simulink library "halout"  (R2021b)
settings: Solver=VariableStepAuto  StartTime=0.0  StopTime=10.0  RelTol=1e-3
undefined symbols (not defined in the file): C_TASK_5MS_S, FALSE, KHAL_CAN1TxReq_flg, KHAL_CAN2TxReq_flg, KHAL_CAN3FD3VCU1toNIDECTxReq_flg, KHAL_CAN3FD3VCU1TxReq_flg, KHAL_CAN3FD3VCU2E2E_flg, KHAL_CAN3FD3VCU2toNIDECE2E_flg, KHAL_CAN3FD3VCU2toNIDECTxReq_flg, KHAL_CAN3FD3VCU2TxReq_flg, KHAL_CAN3TxReq_flg, KHAL_CAN4FD4CE1000E2E_flg, KHAL_CAN4FD4CE1000TxReq_flg, KHAL_CAN4TxReq_flg, KHAL_CAN5TxReq_flg, KHAL_CAN7TxReq_flg, ONE_INT, TRUE, ZERO_INT
libraries: FVT_lib x258, simulink x115
(part 16 of 17)

== system halout/HAL_OUT/CAN4/FD4_CE200_0_0x217/AmbLightColor4 ==
  AmbLightColor4 : Inport
  Data Type Conversion : DataTypeConversion  OutDataTypeStr=uint8  RndMeth=Round
  CAN4_AmbLightColor4 : Outport
  wires:
  Data Type Conversion/1 -> CAN4_AmbLightColor4/1
  AmbLightColor4/1 -> Data Type Conversion/1

== system halout/HAL_OUT/CAN4/FD4_CE200_0_0x217/AmbLightColor5 ==
  AmbLightColor5 : Inport
  Data Type Conversion : DataTypeConversion  OutDataTypeStr=uint8  RndMeth=Round
  CAN4_AmbLightColor5 : Outport
  wires:
  Data Type Conversion/1 -> CAN4_AmbLightColor5/1
  AmbLightColor5/1 -> Data Type Conversion/1

== system halout/HAL_OUT/CAN4/FD4_CE200_0_0x217/AmbLightColor6 ==
  AmbLightColor6 : Inport
  Data Type Conversion : DataTypeConversion  OutDataTypeStr=uint8  RndMeth=Round
  CAN4_AmbLightColor6 : Outport
  wires:
  Data Type Conversion/1 -> CAN4_AmbLightColor6/1
  AmbLightColor6/1 -> Data Type Conversion/1

== system halout/HAL_OUT/CAN4/FD4_CE200_0_0x217/BCMBuzzerReq ==
  BCMBuzzerReq : Inport
  Data Type Conversion : DataTypeConversion  OutDataTypeStr=uint8  RndMeth=Round
  CAN4_BCM_Buzzer_Req : Outport
  wires:
  Data Type Conversion/1 -> CAN4_BCM_Buzzer_Req/1
  BCMBuzzerReq/1 -> Data Type Conversion/1

== system halout/HAL_OUT/CAN4/FD4_CE200_0_0x217/FDCBCMATCtrlCmd ==
  FDCBCMATCtrlCmd : Inport
  Data Type Conversion : DataTypeConversion  OutDataTypeStr=uint8  RndMeth=Round
  CAN4_FDC_BCM_ATCtrl_Cmd : Outport
  wires:
  Data Type Conversion/1 -> CAN4_FDC_BCM_ATCtrl_Cmd/1
  FDCBCMATCtrlCmd/1 -> Data Type Conversion/1

== system halout/HAL_OUT/CAN4/FD4_CE200_0_0x217/FDCBCMDimSw ==
  FDCBCMDimSw : Inport
  Data Type Conversion : DataTypeConversion  OutDataTypeStr=uint8  RndMeth=Round
  CAN4_FDC_BCM_DimSw : Outport
  wires:
  Data Type Conversion/1 -> CAN4_FDC_BCM_DimSw/1
  FDCBCMDimSw/1 -> Data Type Conversion/1

== system halout/HAL_OUT/CAN4/FD4_CE200_0_0x217/FDCBCMFWasSwSta ==
  FDCBCMFWasSwSta : Inport
  Data Type Conversion : DataTypeConversion  OutDataTypeStr=uint8  RndMeth=Round
  CAN4_FDC_BCM_FWasSw_Sta : Outport
  wires:
  Data Type Conversion/1 -> CAN4_FDC_BCM_FWasSw_Sta/1
  FDCBCMFWasSwSta/1 -> Data Type Conversion/1

== system halout/HAL_OUT/CAN4/FD4_CE200_0_0x217/FDCBCMFWipSwSta ==
  FDCBCMFWipSwSta : Inport
  Data Type Conversion : DataTypeConversion  OutDataTypeStr=uint8  RndMeth=Round
  CAN4_FDC_BCM_FWipSw_Sta : Outport
  wires:
  Data Type Conversion/1 -> CAN4_FDC_BCM_FWipSw_Sta/1
  FDCBCMFWipSwSta/1 -> Data Type Conversion/1

== system halout/HAL_OUT/CAN4/FD4_CE200_0_0x217/FDCBCMHazardINDCmd ==
  FDCBCMHazardINDCmd : Inport
  Data Type Conversion : DataTypeConversion  OutDataTypeStr=uint8  RndMeth=Round
  CAN4_FDC_BCM_HazardIND_Cmd : Outport
  wires:
  Data Type Conversion/1 -> CAN4_FDC_BCM_HazardIND_Cmd/1
  FDCBCMHazardINDCmd/1 -> Data Type Conversion/1

== system halout/HAL_OUT/CAN4/FD4_CE200_0_0x217/FDCBCMLockAlarmCmd ==
  FDCBCMLockAlarmCmd : Inport
  Data Type Conversion : DataTypeConversion  OutDataTypeStr=uint8  RndMeth=Round
  CAN4_FDC_BCM_LockAlarm_Cmd : Outport
  wires:
  Data Type Conversion/1 -> CAN4_FDC_BCM_LockAlarm_Cmd/1
  FDCBCMLockAlarmCmd/1 -> Data Type Conversion/1

== system halout/HAL_OUT/CAN4/FD4_CE200_0_0x217/FDCBCMOutModeCmd ==
  FDCBCMOutModeCmd : Inport
  Data Type Conversion : DataTypeConversion  OutDataTypeStr=uint8  RndMeth=Round
  CAN4_FDC_BCM_OutMode_Cmd : Outport
  wires:
  Data Type Conversion/1 -> CAN4_FDC_BCM_OutMode_Cmd/1
  FDCBCMOutModeCmd/1 -> Data Type Conversion/1

== system halout/HAL_OUT/CAN4/FD4_CE200_0_0x217/FDCBCMPTGOpenHeightSta ==
  FDCBCMPTGOpenHeightSta : Inport
  Data Type Conversion : DataTypeConversion  OutDataTypeStr=uint8  RndMeth=Round
  CAN4_FDC_BCM_PTGOpenHeight_Sta : Outport
  wires:
  Data Type Conversion/1 -> CAN4_FDC_BCM_PTGOpenHeight_Sta/1
  FDCBCMPTGOpenHeightSta/1 -> Data Type Conversion/1

== system halout/HAL_OUT/CAN4/FD4_CE200_0_0x217/FDCBCMPassSWSta ==
  FDCBCMPassSWSta : Inport
  Data Type Conversion : DataTypeConversion  OutDataTypeStr=uint8  RndMeth=Round
  CAN4_FDC_BCM_PassSW_Sta : Outport
  wires:
  Data Type Conversion/1 -> CAN4_FDC_BCM_PassSW_Sta/1
  FDCBCMPassSWSta/1 -> Data Type Conversion/1

== system halout/HAL_OUT/CAN4/FD4_CE200_0_0x217/FDCBCMTurnSwSta ==
  FDCBCMTurnSwSta : Inport
  Data Type Conversion : DataTypeConversion  OutDataTypeStr=uint8  RndMeth=Round
  CAN4_FDC_BCM_TurnSw_Sta : Outport
  wires:
  Data Type Conversion/1 -> CAN4_FDC_BCM_TurnSw_Sta/1
  FDCBCMTurnSwSta/1 -> Data Type Conversion/1

== system halout/HAL_OUT/CAN4/FD4_CE200_0_0x217/FDCBCMTurnSwTSetStaSta ==
  FDCBCMTurnSwTSetStaSta : Inport
  Data Type Conversion : DataTypeConversion  OutDataTypeStr=uint8  RndMeth=Round
  CAN4_FDC_BCM_TurnSwTSetSta_Sta : Outport
  wires:
  Data Type Conversion/1 -> CAN4_FDC_BCM_TurnSwTSetSta_Sta/1
  FDCBCMTurnSwTSetStaSta/1 -> Data Type Conversion/1

== system halout/HAL_OUT/CAN4/FD4_CE200_0_0x217/FDCBCMUserHeightSetSta ==
  FDCBCMUserHeightSetSta : Inport
  Data Type Conversion : DataTypeConversion  OutDataTypeStr=uint16  RndMeth=Round
  CAN4_FDC_BCM_UserHeightSet_Sta : Outport
  wires:
  Data Type Conversion/1 -> CAN4_FDC_BCM_UserHeightSet_Sta/1
  FDCBCMUserHeightSetSta/1 -> Data Type Conversion/1

== system halout/HAL_OUT/CAN4/FD4_CE200_0_0x217/FDCBCMUserNowSta ==
  FDCBCMUserNowSta : Inport
  Data Type Conversion : DataTypeConversion  OutDataTypeStr=uint8  RndMeth=Round
  CAN4_FDC_BCM_UserNow_Sta : Outport
  wires:
  Data Type Conversion/1 -> CAN4_FDC_BCM_UserNow_Sta/1
  FDCBCMUserNowSta/1 -> Data Type Conversion/1

== system halout/HAL_OUT/CAN4/FD4_CE200_0_0x217/FDCDKCCommandToBCMCmd ==
  FDCDKCCommandToBCMCmd : Inport
  Data Type Conversion : DataTypeConversion  OutDataTypeStr=uint8  RndMeth=Round
  CAN4_FDC_DKC_CommandToBCM_Cmd : Outport
  wires:
  Data Type Conversion/1 -> CAN4_FDC_DKC_CommandToBCM_Cmd/1
  FDCDKCCommandToBCMCmd/1 -> Data Type Conversion/1

== system halout/HAL_OUT/CAN4/FD4_CE200_0_0x217/FDCDKCDKeyAreaPESta ==
  FDCDKCDKeyAreaPESta : Inport
  Data Type Conversion : DataTypeConversion  OutDataTypeStr=uint8  RndMeth=Round
  CAN4_FDC_DKC_DKeyAreaPE_Sta : Outport
  wires:
  Data Type Conversion/1 -> CAN4_FDC_DKC_DKeyAreaPE_Sta/1
  FDCDKCDKeyAreaPESta/1 -> Data Type Conversion/1

== system halout/HAL_OUT/CAN4/FD4_CE200_0_0x217/FDCDKCSPTGDetCmd ==
  FDCDKCSPTGDetCmd : Inport
  Data Type Conversion : DataTypeConversion  OutDataTypeStr=uint8  RndMeth=Round
  CAN4_FDC_DKC_SPTGDet_Cmd : Outport
  wires:
  Data Type Conversion/1 -> CAN4_FDC_DKC_SPTGDet_Cmd/1
  FDCDKCSPTGDetCmd/1 -> Data Type Conversion/1

== system halout/HAL_OUT/CAN4/FD4_CE200_0_0x217/FDCDKCSPTGOpenCmd ==
  FDCDKCSPTGOpenCmd : Inport
  Data Type Conversion : DataTypeConversion  OutDataTypeStr=uint8  RndMeth=Round
  CAN4_FDC_DKC_SPTGOpen_Cmd : Outport
  wires:
  Data Type Conversion/1 -> CAN4_FDC_DKC_SPTGOpen_Cmd/1
  FDCDKCSPTGOpenCmd/1 -> Data Type Conversion/1

== system halout/HAL_OUT/CAN4/FD4_CE200_0_0x217/FDCEChrgSWSta ==
  FDCEChrgSWSta : Inport
  Data Type Conversion : DataTypeConversion  OutDataTypeStr=uint8  RndMeth=Round
  CAN4_FDC_EChrg_SW_Sta : Outport
  wires:
  Data Type Conversion/1 -> CAN4_FDC_EChrg_SW_Sta/1
  FDCEChrgSWSta/1 -> Data Type Conversion/1

== system halout/HAL_OUT/CAN4/FD4_CE200_0_0x217/FDCTHCMACTInitialCmd ==
  FDCTHCMACTInitialCmd : Inport
  Data Type Conversion : DataTypeConversion  OutDataTypeStr=uint8  RndMeth=Round
  CAN4_FDC_THCM_ACTInitial_Cmd : Outport
  wires:
  Data Type Conversion/1 -> CAN4_FDC_THCM_ACTInitial_Cmd/1
  FDCTHCMACTInitialCmd/1 -> Data Type Conversion/1

== system halout/HAL_OUT/CAN4/FD4_CE200_0_0x217/FDCTHCMAirIntZ3Sta ==
  FDCTHCMAirIntZ3Sta : Inport
  Data Type Conversion : DataTypeConversion  OutDataTypeStr=uint8  RndMeth=Round
  CAN4_FDC_THCM_AirIntZ3_Sta : Outport
  wires:
  Data Type Conversion/1 -> CAN4_FDC_THCM_AirIntZ3_Sta/1
  FDCTHCMAirIntZ3Sta/1 -> Data Type Conversion/1

== system halout/HAL_OUT/CAN4/FD4_CE200_0_0x217/FDHandleCmd ==
  FDHandleCmd : Inport
  Data Type Conversion : DataTypeConversion  OutDataTypeStr=uint8  RndMeth=Round
  CAN4_FDHandleCmd : Outport
  wires:
  Data Type Conversion/1 -> CAN4_FDHandleCmd/1
  FDHandleCmd/1 -> Data Type Conversion/1

== system halout/HAL_OUT/CAN4/FD4_CE200_0_0x217/FDLHandleLampCmd ==
  FDLHandleLampCmd : Inport
  Data Type Conversion : DataTypeConversion  OutDataTypeStr=uint8  RndMeth=Round
  CAN4_FDLHandleLampCmd : Outport
  wires:
  Data Type Conversion/1 -> CAN4_FDLHandleLampCmd/1
  FDLHandleLampCmd/1 -> Data Type Conversion/1

== system halout/HAL_OUT/CAN4/FD4_CE200_0_0x217/FDRHandleLampCmd ==
  FDRHandleLampCmd : Inport
  Data Type Conversion : DataTypeConversion  OutDataTypeStr=uint8  RndMeth=Round
  CAN4_FDRHandleLampCmd : Outport
  wires:
  Data Type Conversion/1 -> CAN4_FDRHandleLampCmd/1
  FDRHandleLampCmd/1 -> Data Type Conversion/1

== system halout/HAL_OUT/CAN4/FD4_CE200_0_0x217/WelcomeLight ==
  WelcomeLight : Inport
  Data Type Conversion : DataTypeConversion  OutDataTypeStr=uint8  RndMeth=Round
  CAN4_WelcomeLight : Outport
  wires:
  Data Type Conversion/1 -> CAN4_WelcomeLight/1
  WelcomeLight/1 -> Data Type Conversion/1

== system halout/HAL_OUT/CAN4/GW4_CE100_0_0x253/BrkPedalPos ==
  BrkPedalPos : Inport
  Data Type Conversion : DataTypeConversion  OutDataTypeStr=uint8  RndMeth=Round
  convert_out : FVT_lib/hal/convert_out  gain=0.4  offset=0
  CAN4_BrkPedalPos : Outport
  wires:
  Data Type Conversion/1 -> CAN4_BrkPedalPos/1
  convert_out/1 -> Data Type Conversion/1
  BrkPedalPos/1 -> convert_out/1

== system halout/HAL_OUT/CAN4/GW4_CE100_0_0x253/BrkPedalPosSta ==
  BrkPedalPosSta : Inport
  Data Type Conversion : DataTypeConversion  OutDataTypeStr=uint8  RndMeth=Round
  CAN4_BrkPedalPos_Sta : Outport
  wires:
  Data Type Conversion/1 -> CAN4_BrkPedalPos_Sta/1
  BrkPedalPosSta/1 -> Data Type Conversion/1

== system halout/HAL_OUT/CAN4/GW4_CE100_0_0x253/BrkSwSta ==
  BrkSwSta : Inport
  Data Type Conversion : DataTypeConversion  OutDataTypeStr=uint8  RndMeth=Round
  CAN4_BrkSw_Sta : Outport
  wires:
  Data Type Conversion/1 -> CAN4_BrkSw_Sta/1
  BrkSwSta/1 -> Data Type Conversion/1

== system halout/HAL_OUT/CAN4/GW4_CE100_0_0x253/BrkSwV ==
  BrkSwV : Inport
  Data Type Conversion : DataTypeConversion  OutDataTypeStr=uint8  RndMeth=Round
  CAN4_BrkSw_V : Outport
  wires:
  Data Type Conversion/1 -> CAN4_BrkSw_V/1
  BrkSwV/1 -> Data Type Conversion/1

== system halout/HAL_OUT/CAN4/GW4_CE100_0_0x253/FDCPTGinnerSW2 ==
  FDCPTGinnerSW2 : Inport
  Data Type Conversion : DataTypeConversion  OutDataTypeStr=uint8  RndMeth=Round
  CAN4_FDC_PTG_inner_SW_2 : Outport
  wires:
  Data Type Conversion/1 -> CAN4_FDC_PTG_inner_SW_2/1
  FDCPTGinnerSW2/1 -> Data Type Conversion/1

== system halout/HAL_OUT/CAN4/GW4_CE100_0_0x253/LDrvCtrlCmd ==
  LDrvCtrlCmd : Inport
  Data Type Conversion : DataTypeConversion  OutDataTypeStr=uint8  RndMeth=Round
  CAN4_L_Drv_CtrlCmd : Outport
  wires:
  Data Type Conversion/1 -> CAN4_L_Drv_CtrlCmd/1
  LDrvCtrlCmd/1 -> Data Type Conversion/1

== system halout/HAL_OUT/CAN4/GW4_CE100_0_0x253/LPasCtrlCmd ==
  LPasCtrlCmd : Inport
  Data Type Conversion : DataTypeConversion  OutDataTypeStr=uint8  RndMeth=Round
  CAN4_L_Pas_CtrlCmd : Outport
  wires:
  Data Type Conversion/1 -> CAN4_L_Pas_CtrlCmd/1
  LPasCtrlCmd/1 -> Data Type Conversion/1

== system halout/HAL_OUT/CAN4/GW4_CE100_0_0x253/LRLDCtrlCmd ==
  LRLDCtrlCmd : Inport
  Data Type Conversion : DataTypeConversion  OutDataTypeStr=uint8  RndMeth=Round
  CAN4_L_RLD_CtrlCmd : Outport
  wires:
  Data Type Conversion/1 -> CAN4_L_RLD_CtrlCmd/1
  LRLDCtrlCmd/1 -> Data Type Conversion/1

== system halout/HAL_OUT/CAN4/GW4_CE100_0_0x253/LRRDCtrlCmd ==
  LRRDCtrlCmd : Inport
  Data Type Conversion : DataTypeConversion  OutDataTypeStr=uint8  RndMeth=Round
  CAN4_L_RRD_CtrlCmd : Outport
  wires:
  Data Type Conversion/1 -> CAN4_L_RRD_CtrlCmd/1
  LRRDCtrlCmd/1 -> Data Type Conversion/1

== system halout/HAL_OUT/CAN4/GW4_CE100_0_0x253/MCPressure ==
  MCPressure : Inport
  Data Type Conversion : DataTypeConversion  OutDataTypeStr=uint16  RndMeth=Round
  convert_out : FVT_lib/hal/convert_out  gain=0.1  offset=-9.7
  CAN4_MCPressure : Outport
  wires:
  Data Type Conversion/1 -> CAN4_MCPressure/1
  convert_out/1 -> Data Type Conversion/1
  MCPressure/1 -> convert_out/1

== system halout/HAL_OUT/CAN4/GW4_CE100_0_0x253/MCPressureV ==
  MCPressureV : Inport
  Data Type Conversion : DataTypeConversion  OutDataTypeStr=uint8  RndMeth=Round
  CAN4_MCPressure_V : Outport
  wires:
  Data Type Conversion/1 -> CAN4_MCPressure_V/1
  MCPressureV/1 -> Data Type Conversion/1

== system halout/HAL_OUT/CAN4/GW4_CE100_0_0x253/VehSpeed ==
  VehSpeed : Inport
  Data Type Conversion : DataTypeConversion  OutDataTypeStr=uint16  RndMeth=Round
  convert_out : FVT_lib/hal/convert_out  gain=0.125  offset=0
  CAN4_VehSpeed : Outport
  wires:
  Data Type Conversion/1 -> CAN4_VehSpeed/1
  convert_out/1 -> Data Type Conversion/1
  VehSpeed/1 -> convert_out/1

== system halout/HAL_OUT/CAN5/FD5_CE100_0_0x118/AllDoorSW ==
  AllDoorSW : Inport
  Data Type Conversion : DataTypeConversion  OutDataTypeStr=uint8  RndMeth=Round
  CAN5_AllDoorSW : Outport
  wires:
  Data Type Conversion/1 -> CAN5_AllDoorSW/1
  AllDoorSW/1 -> Data Type Conversion/1

== system halout/HAL_OUT/CAN5/FD5_CE100_0_0x118/AntitheftSta ==
  AntitheftSta : Inport
  Data Type Conversion : DataTypeConversion  OutDataTypeStr=uint8  RndMeth=Round
  CAN5_AntitheftSta : Outport
  wires:
  Data Type Conversion/1 -> CAN5_AntitheftSta/1
  AntitheftSta/1 -> Data Type Conversion/1

== system halout/HAL_OUT/CAN5/FD5_CE100_0_0x118/BCMDoorLockSta ==
  BCMDoorLockSta : Inport
  Data Type Conversion : DataTypeConversion  OutDataTypeStr=uint8  RndMeth=Round
  CAN5_BCM_DoorLock_Sta : Outport
  wires:
  Data Type Conversion/1 -> CAN5_BCM_DoorLock_Sta/1
  BCMDoorLockSta/1 -> Data Type Conversion/1

== system halout/HAL_OUT/CAN5/FD5_CE100_0_0x118/CCUACLampSts ==
  CCUACLampSts : Inport
  Data Type Conversion : DataTypeConversion  OutDataTypeStr=uint8  RndMeth=Round
  CAN5_CCU_ACLampSts : Outport
  wires:
  Data Type Conversion/1 -> CAN5_CCU_ACLampSts/1
  CCUACLampSts/1 -> Data Type Conversion/1

== system halout/HAL_OUT/CAN5/FD5_CE100_0_0x118/CCUCbnPreACWkSts ==
  CCUCbnPreACWkSts : Inport
  Data Type Conversion : DataTypeConversion  OutDataTypeStr=uint8  RndMeth=Round
  CAN5_CCU_CbnPreACWkSts : Outport
  wires:
  Data Type Conversion/1 -> CAN5_CCU_CbnPreACWkSts/1
  CCUCbnPreACWkSts/1 -> Data Type Conversion/1

== system halout/HAL_OUT/CAN5/FD5_CE100_0_0x118/CCUCbnPreEstimdTi ==
  CCUCbnPreEstimdTi : Inport
  Data Type Conversion : DataTypeConversion  OutDataTypeStr=uint8  RndMeth=Round
  CAN5_CCU_CbnPreEstimdTi : Outport
  wires:
  Data Type Conversion/1 -> CAN5_CCU_CbnPreEstimdTi/1
  CCUCbnPreEstimdTi/1 -> Data Type Conversion/1

== system halout/HAL_OUT/CAN5/FD5_CE100_0_0x118/CCUCbnPreSts ==
  CCUCbnPreSts : Inport
  Data Type Conversion : DataTypeConversion  OutDataTypeStr=uint8  RndMeth=Round
  CAN5_CCU_CbnPreSts : Outport
  wires:
  Data Type Conversion/1 -> CAN5_CCU_CbnPreSts/1
  CCUCbnPreSts/1 -> Data Type Conversion/1

== system halout/HAL_OUT/CAN5/FD5_CE100_0_0x118/FDTBOXDTCDataErr ==
  FDTBOXDTCDataErr : Inport
  Data Type Conversion : DataTypeConversion  OutDataTypeStr=uint8  RndMeth=Round
  CAN5_FD_TBOX_DTCData_Err : Outport
  wires:
  Data Type Conversion/1 -> CAN5_FD_TBOX_DTCData_Err/1
  FDTBOXDTCDataErr/1 -> Data Type Conversion/1

== system halout/HAL_OUT/CAN5/FD5_CE100_0_0x118/FDTBOXDTCDataSta ==
  FDTBOXDTCDataSta : Inport
  Data Type Conversion : DataTypeConversion  OutDataTypeStr=uint8  RndMeth=Round
  CAN5_FD_TBOX_DTCData_Sta : Outport
  wires:
  Data Type Conversion/1 -> CAN5_FD_TBOX_DTCData_Sta/1
  FDTBOXDTCDataSta/1 -> Data Type Conversion/1

== system halout/HAL_OUT/CAN5/FD5_CE100_0_0x118/FDTBOXVehDataErr ==
  FDTBOXVehDataErr : Inport
  Data Type Conversion : DataTypeConversion  OutDataTypeStr=uint8  RndMeth=Round
  CAN5_FD_TBOX_VehData_Err : Outport
  wires:
  Data Type Conversion/1 -> CAN5_FD_TBOX_VehData_Err/1
  FDTBOXVehDataErr/1 -> Data Type Conversion/1

== system halout/HAL_OUT/CAN5/FD5_CE100_0_0x118/FDTBOXVehDataSta ==
  FDTBOXVehDataSta : Inport
  Data Type Conversion : DataTypeConversion  OutDataTypeStr=uint8  RndMeth=Round
  CAN5_FD_TBOX_VehData_Sta : Outport
  wires:
  Data Type Conversion/1 -> CAN5_FD_TBOX_VehData_Sta/1
  FDTBOXVehDataSta/1 -> Data Type Conversion/1

== system halout/HAL_OUT/CAN5/FD5_CE100_0_0x118/HoodSW ==
  HoodSW : Inport
  Data Type Conversion : DataTypeConversion  OutDataTypeStr=uint8  RndMeth=Round
  CAN5_HoodSW : Outport
  wires:
  Data Type Conversion/1 -> CAN5_HoodSW/1
  HoodSW/1 -> Data Type Conversion/1

== system halout/HAL_OUT/CAN5/FD5_CE100_0_0x118/LowSOCWarn ==
  LowSOCWarn : Inport
  Data Type Conversion : DataTypeConversion  OutDataTypeStr=uint8  RndMeth=Round
  CAN5_LowSOCWarn : Outport
  wires:
  Data Type Conversion/1 -> CAN5_LowSOCWarn/1
  LowSOCWarn/1 -> Data Type Conversion/1

== system halout/HAL_OUT/CAN5/FD5_CE100_0_0x118/PwrSta ==
  PwrSta : Inport
  Data Type Conversion : DataTypeConversion  OutDataTypeStr=uint8  RndMeth=Round
  CAN5_PwrSta : Outport
  wires:
  Data Type Conversion/1 -> CAN5_PwrSta/1
  PwrSta/1 -> Data Type Conversion/1

== system halout/HAL_OUT/CAN5/FD5_CE100_0_0x118/ReVehThdChkSta ==
  ReVehThdChkSta : Inport
  Data Type Conversion : DataTypeConversion  OutDataTypeStr=uint8  RndMeth=Round
  CAN5_Re_VehThdChkSta : Outport
  wires:
  Data Type Conversion/1 -> CAN5_Re_VehThdChkSta/1
  ReVehThdChkSta/1 -> Data Type Conversion/1

== system halout/HAL_OUT/CAN5/FD5_CE100_0_0x118/ShiftGearPosn ==
  ShiftGearPosn : Inport
  Data Type Conversion : DataTypeConversion  OutDataTypeStr=uint8  RndMeth=Round
  CAN5_ShiftGearPosn : Outport
  wires:
  Data Type Conversion/1 -> CAN5_ShiftGearPosn/1
  ShiftGearPosn/1 -> Data Type Conversion/1

== system halout/HAL_OUT/CAN5/FD5_CE100_0_0x118/TCountSta ==
  TCountSta : Inport
  Data Type Conversion : DataTypeConversion  OutDataTypeStr=uint8  RndMeth=Round
  CAN5_TCountSta : Outport
  wires:
  Data Type Conversion/1 -> CAN5_TCountSta/1
  TCountSta/1 -> Data Type Conversion/1

== system halout/HAL_OUT/CAN5/FD5_CE100_0_0x118/TailgateRemote ==
  TailgateRemote : Inport
  Data Type Conversion : DataTypeConversion  OutDataTypeStr=uint8  RndMeth=Round
  CAN5_TailgateRemote : Outport
  wires:
  Data Type Conversion/1 -> CAN5_TailgateRemote/1
  TailgateRemote/1 -> Data Type Conversion/1

== system halout/HAL_OUT/CAN5/FD5_CE100_0_0x118/TailgateSW ==
  TailgateSW : Inport
  Data Type Conversion : DataTypeConversion  OutDataTypeStr=uint8  RndMeth=Round
  CAN5_Tailgate_SW : Outport
  wires:
  Data Type Conversion/1 -> CAN5_Tailgate_SW/1
  TailgateSW/1 -> Data Type Conversion/1

== system halout/HAL_OUT/CAN5/FD5_CE100_0_0x118/VehMalfunLevel ==
  VehMalfunLevel : Inport
  Data Type Conversion : DataTypeConversion  OutDataTypeStr=uint8  RndMeth=Round
  CAN5_VehMalfunLevel : Outport
  wires:
  Data Type Conversion/1 -> CAN5_VehMalfunLevel/1
  VehMalfunLevel/1 -> Data Type Conversion/1

== system halout/HAL_OUT/CAN5/FD5_Debug1_0x4D0/ID1ALTU ==
  ID1ALTU : Inport
  Data Type Conversion : DataTypeConversion  OutDataTypeStr=uint32  RndMeth=Round
  CAN5_ID1_ALTU : Outport
  wires:
  Data Type Conversion/1 -> CAN5_ID1_ALTU/1
  ID1ALTU/1 -> Data Type Conversion/1

== system halout/HAL_OUT/CAN5/FD5_Debug1_0x4D0/ID1LocALTU ==
  ID1LocALTU : Inport
  Data Type Conversion : DataTypeConversion  OutDataTypeStr=uint8  RndMeth=Round
  CAN5_ID1_Loc_ALTU : Outport
  wires:
  Data Type Conversion/1 -> CAN5_ID1_Loc_ALTU/1
  ID1LocALTU/1 -> Data Type Conversion/1

== system halout/HAL_OUT/CAN5/FD5_Debug1_0x4D0/ID1messageALTU ==
  ID1messageALTU : Inport
  Data Type Conversion : DataTypeConversion  OutDataTypeStr=uint8  RndMeth=Round
  CAN5_ID1_message_ALTU : Outport
  wires:
  Data Type Conversion/1 -> CAN5_ID1_message_ALTU/1
  ID1messageALTU/1 -> Data Type Conversion/1

== system halout/HAL_OUT/CAN5/FD5_Debug1_0x4D0/ID2ALTU ==
  ID2ALTU : Inport
  Data Type Conversion : DataTypeConversion  OutDataTypeStr=uint32  RndMeth=Round
  CAN5_ID2_ALTU : Outport
  wires:
  Data Type Conversion/1 -> CAN5_ID2_ALTU/1
  ID2ALTU/1 -> Data Type Conversion/1

== system halout/HAL_OUT/CAN5/FD5_Debug1_0x4D0/ID2LocALTU ==
  ID2LocALTU : Inport
  Data Type Conversion : DataTypeConversion  OutDataTypeStr=uint8  RndMeth=Round
  CAN5_ID2_Loc_ALTU : Outport
  wires:
  Data Type Conversion/1 -> CAN5_ID2_Loc_ALTU/1
  ID2LocALTU/1 -> Data Type Conversion/1

== system halout/HAL_OUT/CAN5/FD5_Debug1_0x4D0/ID2messageALTU ==
  ID2messageALTU : Inport
  Data Type Conversion : DataTypeConversion  OutDataTypeStr=uint8  RndMeth=Round
  CAN5_ID2_message_ALTU : Outport
  wires:
  Data Type Conversion/1 -> CAN5_ID2_message_ALTU/1
  ID2messageALTU/1 -> Data Type Conversion/1

== system halout/HAL_OUT/CAN5/FD5_Debug1_0x4D0/ID3ALTU ==
  ID3ALTU : Inport
  Data Type Conversion : DataTypeConversion  OutDataTypeStr=uint32  RndMeth=Round
  CAN5_ID3_ALTU : Outport
  wires:
  Data Type Conversion/1 -> CAN5_ID3_ALTU/1
  ID3ALTU/1 -> Data Type Conversion/1

== system halout/HAL_OUT/CAN5/FD5_Debug1_0x4D0/ID3LocALTU ==
  ID3LocALTU : Inport
  Data Type Conversion : DataTypeConversion  OutDataTypeStr=uint8  RndMeth=Round
  CAN5_ID3_Loc_ALTU : Outport
  wires:
  Data Type Conversion/1 -> CAN5_ID3_Loc_ALTU/1
  ID3LocALTU/1 -> Data Type Conversion/1

== system halout/HAL_OUT/CAN5/FD5_Debug1_0x4D0/ID3messageALTU ==
  ID3messageALTU : Inport
  Data Type Conversion : DataTypeConversion  OutDataTypeStr=uint8  RndMeth=Round
  CAN5_ID3_message_ALTU : Outport
  wires:
  Data Type Conversion/1 -> CAN5_ID3_message_ALTU/1
  ID3messageALTU/1 -> Data Type Conversion/1

== system halout/HAL_OUT/CAN5/FD5_Debug1_0x4D0/ID4ALTU ==
  ID4ALTU : Inport
  Data Type Conversion : DataTypeConversion  OutDataTypeStr=uint32  RndMeth=Round
  CAN5_ID4_ALTU : Outport
  wires:
  Data Type Conversion/1 -> CAN5_ID4_ALTU/1
  ID4ALTU/1 -> Data Type Conversion/1

== system halout/HAL_OUT/CAN5/FD5_Debug1_0x4D0/ID4LocALTU ==
  ID4LocALTU : Inport
  Data Type Conversion : DataTypeConversion  OutDataTypeStr=uint8  RndMeth=Round
  CAN5_ID4_Loc_ALTU : Outport
  wires:
  Data Type Conversion/1 -> CAN5_ID4_Loc_ALTU/1
  ID4LocALTU/1 -> Data Type Conversion/1

== system halout/HAL_OUT/CAN5/FD5_Debug1_0x4D0/ID4messageALTU ==
  ID4messageALTU : Inport
  Data Type Conversion : DataTypeConversion  OutDataTypeStr=uint8  RndMeth=Round
  CAN5_ID4_message_ALTU : Outport
  wires:
  Data Type Conversion/1 -> CAN5_ID4_message_ALTU/1
  ID4messageALTU/1 -> Data Type Conversion/1

== system halout/HAL_OUT/CAN5/FD5_Debug1_0x4D0/IDinALTU ==
  IDinALTU : Inport
  Data Type Conversion : DataTypeConversion  OutDataTypeStr=uint32  RndMeth=Round
  CAN5_IDin_ALTU : Outport
  wires:
  Data Type Conversion/1 -> CAN5_IDin_ALTU/1
  IDinALTU/1 -> Data Type Conversion/1

== system halout/HAL_OUT/CAN5/FD5_Debug1_0x4D0/LFSensorMode ==
  LFSensorMode : Inport
  Data Type Conversion : DataTypeConversion  OutDataTypeStr=uint8  RndMeth=Round
  CAN5_LFSensorMode : Outport
  wires:
  Data Type Conversion/1 -> CAN5_LFSensorMode/1
  LFSensorMode/1 -> Data Type Conversion/1

== system halout/HAL_OUT/CAN5/FD5_Debug1_0x4D0/LRSensorMode ==
  LRSensorMode : Inport
  Data Type Conversion : DataTypeConversion  OutDataTypeStr=uint8  RndMeth=Round
  CAN5_LRSensorMode : Outport
  wires:
  Data Type Conversion/1 -> CAN5_LRSensorMode/1
  LRSensorMode/1 -> Data Type Conversion/1

== system halout/HAL_OUT/CAN5/FD5_Debug1_0x4D0/RFFATALTU ==
  RFFATALTU : Inport
  Data Type Conversion : DataTypeConversion  OutDataTypeStr=uint8  RndMeth=Round
  CAN5_RF_FAT_ALTU : Outport
  wires:
  Data Type Conversion/1 -> CAN5_RF_FAT_ALTU/1
  RFFATALTU/1 -> Data Type Conversion/1

== system halout/HAL_OUT/CAN5/FD5_Debug1_0x4D0/RFSensorMode ==
  RFSensorMode : Inport
  Data Type Conversion : DataTypeConversion  OutDataTypeStr=uint8  RndMeth=Round
  CAN5_RFSensorMode : Outport
  wires:
  Data Type Conversion/1 -> CAN5_RFSensorMode/1
  RFSensorMode/1 -> Data Type Conversion/1

== system halout/HAL_OUT/CAN5/FD5_Debug1_0x4D0/RRSensorMode ==
  RRSensorMode : Inport
  Data Type Conversion : DataTypeConversion  OutDataTypeStr=uint8  RndMeth=Round
  CAN5_RRSensorMode : Outport
  wires:
  Data Type Conversion/1 -> CAN5_RRSensorMode/1
  RRSensorMode/1 -> Data Type Conversion/1

== system halout/HAL_OUT/CAN5/FD5_Debug1_0x4D0/S1WheelDebugALTU ==
  S1WheelDebugALTU : Inport
  Data Type Conversion : DataTypeConversion  OutDataTypeStr=uint8  RndMeth=Round
  convert_out : FVT_lib/hal/convert_out  gain=0.5  offset=0
  CAN5_S1WheelDebug_ALTU : Outport
  wires:
  Data Type Conversion/1 -> CAN5_S1WheelDebug_ALTU/1
  convert_out/1 -> Data Type Conversion/1
  S1WheelDebugALTU/1 -> convert_out/1

== system halout/HAL_OUT/CAN5/FD5_Debug1_0x4D0/S2WheelDebugALTU ==
  S2WheelDebugALTU : Inport
  Data Type Conversion : DataTypeConversion  OutDataTypeStr=uint8  RndMeth=Round
  convert_out : FVT_lib/hal/convert_out  gain=0.5  offset=0
  CAN5_S2WheelDebug_ALTU : Outport
  wires:
  Data Type Conversion/1 -> CAN5_S2WheelDebug_ALTU/1
  convert_out/1 -> Data Type Conversion/1
  S2WheelDebugALTU/1 -> convert_out/1

== system halout/HAL_OUT/CAN5/FD5_Debug1_0x4D0/S3WheelDebugALTU ==
  S3WheelDebugALTU : Inport
  Data Type Conversion : DataTypeConversion  OutDataTypeStr=uint8  RndMeth=Round
  convert_out : FVT_lib/hal/convert_out  gain=0.5  offset=0
  CAN5_S3WheelDebug_ALTU : Outport
  wires:
  Data Type Conversion/1 -> CAN5_S3WheelDebug_ALTU/1
  convert_out/1 -> Data Type Conversion/1
  S3WheelDebugALTU/1 -> convert_out/1

== system halout/HAL_OUT/CAN5/FD5_Debug1_0x4D0/S4WheelDebugALTU ==
  S4WheelDebugALTU : Inport
  Data Type Conversion : DataTypeConversion  OutDataTypeStr=uint8  RndMeth=Round
  convert_out : FVT_lib/hal/convert_out  gain=0.5  offset=0
  CAN5_S4WheelDebug_ALTU : Outport
  wires:
  Data Type Conversion/1 -> CAN5_S4WheelDebug_ALTU/1
  convert_out/1 -> Data Type Conversion/1
  S4WheelDebugALTU/1 -> convert_out/1

== system halout/HAL_OUT/CAN5/GW5_CE100_0_0x1C5/BrkSwSta ==
  BrkSwSta : Inport
  Data Type Conversion : DataTypeConversion  OutDataTypeStr=uint8  RndMeth=Round
  CAN5_BrkSw_Sta : Outport
  wires:
  Data Type Conversion/1 -> CAN5_BrkSw_Sta/1
  BrkSwSta/1 -> Data Type Conversion/1

== system halout/HAL_OUT/CAN5/GW5_CE100_0_0x1C5/CrashOutputSts ==
  CrashOutputSts : Inport
  Data Type Conversion : DataTypeConversion  OutDataTypeStr=uint8  RndMeth=Round
  CAN5_CrashOutputSts : Outport
  wires:
  Data Type Conversion/1 -> CAN5_CrashOutputSts/1
  CrashOutputSts/1 -> Data Type Conversion/1

== system halout/HAL_OUT/CAN5/GW5_CE100_0_0x1C5/PTGActiveSta ==
  PTGActiveSta : Inport
  Data Type Conversion : DataTypeConversion  OutDataTypeStr=uint8  RndMeth=Round
  CAN5_PTG_Active_Sta : Outport
  wires:
  Data Type Conversion/1 -> CAN5_PTG_Active_Sta/1
  PTGActiveSta/1 -> Data Type Conversion/1

== system halout/HAL_OUT/CAN5/GW5_CE100_0_0x1C5/PTGExist ==
  PTGExist : Inport
  Data Type Conversion : DataTypeConversion  OutDataTypeStr=uint8  RndMeth=Round
  CAN5_PTG_Exist : Outport
  wires:
  Data Type Conversion/1 -> CAN5_PTG_Exist/1
  PTGExist/1 -> Data Type Conversion/1

== system halout/HAL_OUT/CAN5/GW5_CE100_0_0x1C5/PTGSysSta ==
  PTGSysSta : Inport
  Data Type Conversion : DataTypeConversion  OutDataTypeStr=uint8  RndMeth=Round
  CAN5_PTG_Sys_Sta : Outport
  wires:
  Data Type Conversion/1 -> CAN5_PTG_Sys_Sta/1
  PTGSysSta/1 -> Data Type Conversion/1

== system halout/HAL_OUT/CAN5/GW5_CE100_0_0x1C5/VehSpeed ==
  VehSpeed : Inport
  Data Type Conversion : DataTypeConversion  OutDataTypeStr=uint16  RndMeth=Round
  convert_out : FVT_lib/hal/convert_out  gain=0.125  offset=0
  CAN5_VehSpeed : Outport
  wires:
  Data Type Conversion/1 -> CAN5_VehSpeed/1
  convert_out/1 -> Data Type Conversion/1
  VehSpeed/1 -> convert_out/1

== system halout/HAL_OUT/CAN5/GW5_CE100_0_0x1C5/ZLAPMWinLFOpenedSta ==
  ZLAPMWinLFOpenedSta : Inport
  Data Type Conversion : DataTypeConversion  OutDataTypeStr=uint8  RndMeth=Round
  CAN5_ZL_APM_WinLFOpened_Sta : Outport
  wires:
  Data Type Conversion/1 -> CAN5_ZL_APM_WinLFOpened_Sta/1
  ZLAPMWinLFOpenedSta/1 -> Data Type Conversion/1

== system halout/HAL_OUT/CAN5/GW5_CE100_0_0x1C5/ZLAPMWinLROpenedSta ==
  ZLAPMWinLROpenedSta : Inport
  Data Type Conversion : DataTypeConversion  OutDataTypeStr=uint8  RndMeth=Round
  CAN5_ZL_APM_WinLROpened_Sta : Outport
  wires:
  Data Type Conversion/1 -> CAN5_ZL_APM_WinLROpened_Sta/1
  ZLAPMWinLROpenedSta/1 -> Data Type Conversion/1

== system halout/HAL_OUT/CAN5/GW5_CE100_0_0x1C5/ZRAPMWinRFOpenedSta ==
  ZRAPMWinRFOpenedSta : Inport
  Data Type Conversion : DataTypeConversion  OutDataTypeStr=uint8  RndMeth=Round
  CAN5_ZR_APM_WinRFOpened_Sta : Outport
  wires:
  Data Type Conversion/1 -> CAN5_ZR_APM_WinRFOpened_Sta/1
  ZRAPMWinRFOpenedSta/1 -> Data Type Conversion/1

== system halout/HAL_OUT/CAN5/GW5_CE100_0_0x1C5/ZRAPMWinRROpenedSta ==
  ZRAPMWinRROpenedSta : Inport
  Data Type Conversion : DataTypeConversion  OutDataTypeStr=uint8  RndMeth=Round
  CAN5_ZR_APM_WinRROpened_Sta : Outport
  wires:
  Data Type Conversion/1 -> CAN5_ZR_APM_WinRROpened_Sta/1
  ZRAPMWinRROpenedSta/1 -> Data Type Conversion/1

== system halout/HAL_OUT/CAN5/GW5_CE100_0_0x1C5/ZRPTGActiveSta ==
  ZRPTGActiveSta : Inport
  Data Type Conversion : DataTypeConversion  OutDataTypeStr=uint8  RndMeth=Round
  CAN5_ZR_PTG_Active_Sta : Outport
  wires:
  Data Type Conversion/1 -> CAN5_ZR_PTG_Active_Sta/1
  ZRPTGActiveSta/1 -> Data Type Conversion/1

== system halout/HAL_OUT/CAN5/GW5_CE100_0_0x1C5/ZRPTGExistSta ==
  ZRPTGExistSta : Inport
  Data Type Conversion : DataTypeConversion  OutDataTypeStr=uint8  RndMeth=Round
  CAN5_ZR_PTG_Exist_Sta : Outport
  wires:
  Data Type Conversion/1 -> CAN5_ZR_PTG_Exist_Sta/1
  ZRPTGExistSta/1 -> Data Type Conversion/1

== system halout/HAL_OUT/CAN5/GW5_CE100_0_0x1C5/ZRPTGSysSta ==
  ZRPTGSysSta : Inport
  Data Type Conversion : DataTypeConversion  OutDataTypeStr=uint8  RndMeth=Round
  CAN5_ZR_PTG_Sys_Sta : Outport
  wires:
  Data Type Conversion/1 -> CAN5_ZR_PTG_Sys_Sta/1
  ZRPTGSysSta/1 -> Data Type Conversion/1

== system halout/HAL_OUT/CAN7/FD7_CE100_0_0x18FA05B9/FDCBCMFDDoorOpenSta ==
  FDCBCMFDDoorOpenSta : Inport
  Data Type Conversion : DataTypeConversion  OutDataTypeStr=uint8  RndMeth=Round
  CAN7_FDC_BCM_FDDoorOpen_Sta : Outport
  wires:
  Data Type Conversion/1 -> CAN7_FDC_BCM_FDDoorOpen_Sta/1
  FDCBCMFDDoorOpenSta/1 -> Data Type Conversion/1

== system halout/HAL_OUT/CAN7/FD7_CE100_0_0x18FA05B9/LTurnLP ==
  LTurnLP : Inport
  Data Type Conversion : DataTypeConversion  OutDataTypeStr=uint8  RndMeth=Round
  CAN7_LTurnLP : Outport
  wires:
  Data Type Conversion/1 -> CAN7_LTurnLP/1
  LTurnLP/1 -> Data Type Conversion/1

== system halout/HAL_OUT/CAN7/FD7_CE100_0_0x18FA05B9/RTurnLP ==
  RTurnLP : Inport
  Data Type Conversion : DataTypeConversion  OutDataTypeStr=uint8  RndMeth=Round
  CAN7_RTurnLP : Outport
  wires:
  Data Type Conversion/1 -> CAN7_RTurnLP/1
  RTurnLP/1 -> Data Type Conversion/1

== system halout/HAL_OUT/CAN7/FD7_CE100_1_0xCFFE632/FDCBCMFRClosedoorCmd ==
  FDCBCMFRClosedoorCmd : Inport
  Data Type Conversion : DataTypeConversion  OutDataTypeStr=uint8  RndMeth=Round
  CAN7_FDC_BCM_FRClosedoor_Cmd : Outport
  wires:
  Data Type Conversion/1 -> CAN7_FDC_BCM_FRClosedoor_Cmd/1
  FDCBCMFRClosedoorCmd/1 -> Data Type Conversion/1

== system halout/HAL_OUT/CAN7/FD7_CE100_1_0xCFFE632/FDCBCMFRHaltBrakeSta ==
  FDCBCMFRHaltBrakeSta : Inport
  Data Type Conversion : DataTypeConversion  OutDataTypeStr=uint8  RndMeth=Round
  CAN7_FDC_BCM_FRHaltBrake_Sta : Outport
  wires:
  Data Type Conversion/1 -> CAN7_FDC_BCM_FRHaltBrake_Sta/1
  FDCBCMFRHaltBrakeSta/1 -> Data Type Conversion/1

== system halout/HAL_OUT/CAN7/FD7_CE100_1_0xCFFE632/FDCBCMFROpenClosePBCmd ==
  FDCBCMFROpenClosePBCmd : Inport
  Data Type Conversion : DataTypeConversion  OutDataTypeStr=uint8  RndMeth=Round
  CAN7_FDC_BCM_FROpenClosePB_Cmd : Outport
  wires:
  Data Type Conversion/1 -> CAN7_FDC_BCM_FROpenClosePB_Cmd/1
  FDCBCMFROpenClosePBCmd/1 -> Data Type Conversion/1

== system halout/HAL_OUT/CAN7/FD7_CE100_1_0xCFFE632/FDCBCMFROpendoorCmd ==
  FDCBCMFROpendoorCmd : Inport
  Data Type Conversion : DataTypeConversion  OutDataTypeStr=uint8  RndMeth=Round
  CAN7_FDC_BCM_FROpendoor_Cmd : Outport
  wires:
  Data Type Conversion/1 -> CAN7_FDC_BCM_FROpendoor_Cmd/1
  FDCBCMFROpendoorCmd/1 -> Data Type Conversion/1

== system halout/HAL_OUT/CAN7/FD7_CE100_1_0xCFFE632/FDCBCMPosLampCmd ==
  FDCBCMPosLampCmd : Inport
  Data Type Conversion : DataTypeConversion  OutDataTypeStr=uint8  RndMeth=Round
  CAN7_FDC_BCM_PosLamp_Cmd : Outport
  wires:
  Data Type Conversion/1 -> CAN7_FDC_BCM_PosLamp_Cmd/1
  FDCBCMPosLampCmd/1 -> Data Type Conversion/1

== system halout/HAL_OUT/CAN7/FD7_CE100_1_0xCFFE632/FDCFRDisIntEmCmd ==
  FDCFRDisIntEmCmd : Inport
  Data Type Conversion : DataTypeConversion  OutDataTypeStr=uint8  RndMeth=Round
  CAN7_FDC_FRDisIntEm_Cmd : Outport
  wires:
  Data Type Conversion/1 -> CAN7_FDC_FRDisIntEm_Cmd/1
  FDCFRDisIntEmCmd/1 -> Data Type Conversion/1

== system halout/HAL_OUT/CAN3/FD3_VCU2_0x153/CRC8_IfAction_Tx/If Action Subsystem ==
  Byte1 : Inport
  Action Port : ActionPort
  CRC8_Caculation : Subsystem
      mask help: MeasumentTrigerEvent
      mask Display: fprintf('CRC8');
  CRC8_Result : Outport
  wires:
  CRC8_Caculation/1(CRCout) -> CRC8_Result/1
  Byte1/1 -> CRC8_Caculation/1(MsgData)

== system halout/HAL_OUT/CAN3/FD3_VCU2_0x153/CRC8_IfAction_Tx/If Action Subsystem1 ==
  CAN_E2E_ID1 : Inport
  CAN_E2E_ID2 : Inport  Port=2
  Byte1 : Inport  Port=3
  Action Port : ActionPort
  CRC8_E2EProfile1 : Subsystem
      mask help: MeasumentTrigerEvent
      mask Display: fprintf('CRC8_E2EProfile1');
  Mux2 : Mux  Inputs=3
  CRC8_E2EResult : Outport
  wires:
  Mux2/1 -> CRC8_E2EProfile1/1(MsgData)
  CAN_E2E_ID1/1 -> Mux2/1
  CAN_E2E_ID2/1 -> Mux2/2
  Byte1/1 -> Mux2/3
  CRC8_E2EProfile1/1(CRCout) -> CRC8_E2EResult/1

== system halout/HAL_OUT/CAN3/FD3_VCU2_toNIDEC_0x154/CRC8_IfAction_Tx/If Action Subsystem ==
  Byte1 : Inport
  Action Port : ActionPort
  CRC8_Caculation : Subsystem
      mask help: MeasumentTrigerEvent
      mask Display: fprintf('CRC8');
  CRC8_Result : Outport
  wires:
  CRC8_Caculation/1(CRCout) -> CRC8_Result/1
  Byte1/1 -> CRC8_Caculation/1(MsgData)

== system halout/HAL_OUT/CAN3/FD3_VCU2_toNIDEC_0x154/CRC8_IfAction_Tx/If Action Subsystem1 ==
  CAN_E2E_ID1 : Inport
  CAN_E2E_ID2 : Inport  Port=2
  Byte1 : Inport  Port=3
  Action Port : ActionPort
  CRC8_E2EProfile1 : Subsystem
      mask help: MeasumentTrigerEvent
      mask Display: fprintf('CRC8_E2EProfile1');
  Mux2 : Mux  Inputs=3
  CRC8_E2EResult : Outport
  wires:
  Mux2/1 -> CRC8_E2EProfile1/1(MsgData)
  CAN_E2E_ID1/1 -> Mux2/1
  CAN_E2E_ID2/1 -> Mux2/2
  Byte1/1 -> Mux2/3
  CRC8_E2EProfile1/1(CRCout) -> CRC8_E2EResult/1

== system halout/HAL_OUT/CAN4/FD4_CE100_0_0x116/CRC8_IfAction_Tx/If Action Subsystem ==
  Byte1 : Inport
  Action Port : ActionPort
  CRC8_Caculation : Subsystem
      mask help: MeasumentTrigerEvent
      mask Display: fprintf('CRC8');
  CRC8_Result : Outport
  wires:
  CRC8_Caculation/1(CRCout) -> CRC8_Result/1
  Byte1/1 -> CRC8_Caculation/1(MsgData)

== system halout/HAL_OUT/CAN4/FD4_CE100_0_0x116/CRC8_IfAction_Tx/If Action Subsystem1 ==
  CAN_E2E_ID1 : Inport
  CAN_E2E_ID2 : Inport  Port=2
  Byte1 : Inport  Port=3
  Action Port : ActionPort
  CRC8_E2EProfile1 : Subsystem
      mask help: MeasumentTrigerEvent
      mask Display: fprintf('CRC8_E2EProfile1');
  Mux2 : Mux  Inputs=3
  CRC8_E2EResult : Outport
  wires:
  Mux2/1 -> CRC8_E2EProfile1/1(MsgData)
  CAN_E2E_ID1/1 -> Mux2/1
  CAN_E2E_ID2/1 -> Mux2/2
  Byte1/1 -> Mux2/3
  CRC8_E2EProfile1/1(CRCout) -> CRC8_E2EResult/1

== system halout/HAL_OUT/CAN3/FD3_VCU2_0x153/CRC8_IfAction_Tx/If Action Subsystem/CRC8_Caculation ==
  MsgData : Inport
  Data Type Conversion3 : DataTypeConversion  OutDataTypeStr=uint8
  Data Type Conversion4 : DataTypeConversion  OutDataTypeStr=uint8
  MATLAB Function : MATLAB Function  TreatAsAtomicUnit=on
  CRCout : Outport
  wires:
  Data Type Conversion4/1 -> CRCout/1
  MATLAB Function/1(CRC_Out) -> Data Type Conversion4/1
  Data Type Conversion3/1 -> MATLAB Function/1(msg_raw)
  MsgData/1 -> Data Type Conversion3/1

== system halout/HAL_OUT/CAN3/FD3_VCU2_0x153/CRC8_IfAction_Tx/If Action Subsystem1/CRC8_E2EProfile1 ==
  MsgData : Inport
  Data Type Conversion3 : DataTypeConversion  OutDataTypeStr=uint8
  Data Type Conversion4 : DataTypeConversion  OutDataTypeStr=uint8
  MATLAB Function : MATLAB Function  TreatAsAtomicUnit=on
  CRCout : Outport
  wires:
  MsgData/1 -> Data Type Conversion3/1
  Data Type Conversion3/1 -> MATLAB Function/1(msg_raw)
  MATLAB Function/1(CRC_Out) -> Data Type Conversion4/1
  Data Type Conversion4/1 -> CRCout/1

== system halout/HAL_OUT/CAN3/FD3_VCU2_toNIDEC_0x154/CRC8_IfAction_Tx/If Action Subsystem/CRC8_Caculation ==
  MsgData : Inport
  Data Type Conversion3 : DataTypeConversion  OutDataTypeStr=uint8
  Data Type Conversion4 : DataTypeConversion  OutDataTypeStr=uint8
  MATLAB Function : MATLAB Function  TreatAsAtomicUnit=on
  CRCout : Outport
  wires:
  Data Type Conversion4/1 -> CRCout/1
  MATLAB Function/1(CRC_Out) -> Data Type Conversion4/1
  Data Type Conversion3/1 -> MATLAB Function/1(msg_raw)
  MsgData/1 -> Data Type Conversion3/1

== system halout/HAL_OUT/CAN3/FD3_VCU2_toNIDEC_0x154/CRC8_IfAction_Tx/If Action Subsystem1/CRC8_E2EProfile1 ==
  MsgData : Inport
  Data Type Conversion3 : DataTypeConversion  OutDataTypeStr=uint8
  Data Type Conversion4 : DataTypeConversion  OutDataTypeStr=uint8
  MATLAB Function : MATLAB Function  TreatAsAtomicUnit=on
  CRCout : Outport
  wires:
  MsgData/1 -> Data Type Conversion3/1
  Data Type Conversion3/1 -> MATLAB Function/1(msg_raw)
  MATLAB Function/1(CRC_Out) -> Data Type Conversion4/1
  Data Type Conversion4/1 -> CRCout/1

== system halout/HAL_OUT/CAN4/FD4_CE100_0_0x116/CRC8_IfAction_Tx/If Action Subsystem/CRC8_Caculation ==
  MsgData : Inport
  Data Type Conversion3 : DataTypeConversion  OutDataTypeStr=uint8
  Data Type Conversion4 : DataTypeConversion  OutDataTypeStr=uint8
  MATLAB Function : MATLAB Function  TreatAsAtomicUnit=on
  CRCout : Outport
  wires:
  Data Type Conversion4/1 -> CRCout/1
  MATLAB Function/1(CRC_Out) -> Data Type Conversion4/1
  Data Type Conversion3/1 -> MATLAB Function/1(msg_raw)
  MsgData/1 -> Data Type Conversion3/1

== system halout/HAL_OUT/CAN4/FD4_CE100_0_0x116/CRC8_IfAction_Tx/If Action Subsystem1/CRC8_E2EProfile1 ==
  MsgData : Inport
  Data Type Conversion3 : DataTypeConversion  OutDataTypeStr=uint8
  Data Type Conversion4 : DataTypeConversion  OutDataTypeStr=uint8
  MATLAB Function : MATLAB Function  TreatAsAtomicUnit=on
  CRCout : Outport
  wires:
  MsgData/1 -> Data Type Conversion3/1
  Data Type Conversion3/1 -> MATLAB Function/1(msg_raw)
  MATLAB Function/1(CRC_Out) -> Data Type Conversion4/1
  Data Type Conversion4/1 -> CRCout/1

== stateflow chart halout/HAL_OUT/CAN3/FD3_VCU1_Tx/Chart ==
  state TrigCounter
    en:
    counter = 0;
    counter++;
    (default) -> (junction 5)
    TrigCounter -> (junction 5) : {
        | counter++;
        | TxTrigger = FALSE;
        | CycleTriggerred = FALSE;
        | }
    (junction 5) -> (junction 6) [order 1] : [TxReq && (counter %% CycleCnt) == 0]
    (junction 5) -> (junction 7) [order 2]
    (junction 6) -> (junction 8) : {
        | TxTrigger = TRUE;
        | counter = 0;
        | CycleTriggerred =TRUE;
        | }
    (junction 8) -> (junction 7)
    (junction 7) -> (junction 34)
    (junction 34) -> (junction 38) [order 1] : [TxReq && EventReq && !CycleTriggerred]
    (junction 34) -> (junction 36) [order 2]
    (junction 38) -> (junction 40) : {
        | TxTrigger = TRUE;
        | }
    (junction 40) -> (junction 36)
    (junction 36) -> (junction 21)
    (junction 21) -> (junction 23) [order 1] : [ !TxReq]
    (junction 21) -> (junction 22) [order 2]
    (junction 23) -> (junction 20) : {
        | counter = 0;
        | }
    (junction 20) -> (junction 22)
    (junction 22) -> (junction 31)
  data: TxReq input; EventReq input; CycleCnt input; counter local uint16; CycleTriggerred local boolean; FALSE parameter; TRUE parameter; TxTrigger output double

== stateflow chart halout/HAL_OUT/CAN3/FD3_VCU1_toNIDEC_Tx/Chart ==
  state TrigCounter
    en:
    counter = 0;
    counter++;
    (default) -> (junction 5)
    TrigCounter -> (junction 5) : {
        | counter++;
        | TxTrigger = FALSE;
        | CycleTriggerred = FALSE;
        | }
    (junction 5) -> (junction 6) [order 1] : [TxReq && (counter %% CycleCnt) == 0]
    (junction 5) -> (junction 7) [order 2]
    (junction 6) -> (junction 8) : {
        | TxTrigger = TRUE;
        | counter = 0;
        | CycleTriggerred =TRUE;
        | }
    (junction 8) -> (junction 7)
    (junction 7) -> (junction 34)
    (junction 34) -> (junction 38) [order 1] : [TxReq && EventReq && !CycleTriggerred]
    (junction 34) -> (junction 36) [order 2]
    (junction 38) -> (junction 40) : {
        | TxTrigger = TRUE;
        | }
    (junction 40) -> (junction 36)
    (junction 36) -> (junction 21)
    (junction 21) -> (junction 23) [order 1] : [ !TxReq]
    (junction 21) -> (junction 22) [order 2]
    (junction 23) -> (junction 20) : {
        | counter = 0;
        | }
    (junction 20) -> (junction 22)
    (junction 22) -> (junction 31)
  data: TxReq input; EventReq input; CycleCnt input; counter local uint16; CycleTriggerred local boolean; FALSE parameter; TRUE parameter; TxTrigger output double

== stateflow chart halout/HAL_OUT/CAN3/FD3_VCU2_Tx/Chart ==
  state TrigCounter
    en:
    counter = 0;
    counter++;
    (default) -> (junction 5)
    TrigCounter -> (junction 5) : {
        | counter++;
        | }
    (junction 5) -> (junction 6) [order 1] : [TxReq && (counter %% CycleCnt) == 0]
    (junction 5) -> (junction 7) [order 2]
    (junction 6) -> (junction 8) : {
        | TxTrigger;
        | counter = 0;
        | }
    (junction 8) -> (junction 7)
    (junction 7) -> (junction 34)
    (junction 34) -> (junction 33) [order 1] : [ !TxReq]
    (junction 34) -> (junction 35) [order 2]
    (junction 33) -> (junction 36) : {
        | counter = 0;
        | }
    (junction 36) -> (junction 35)
    (junction 35) -> (junction 44)
  data: TxReq input; CycleCnt input; counter local uint16
  events: TxTrigger output FUNCTION_CALL_EVENT

== matlab function halout/HAL_OUT/CAN3/FD3_VCU2_0x153/CRC8_IfAction_Tx/If Action Subsystem1/CRC8_E2EProfile1/MATLAB Function ==
  data: msg_raw input; CRC_Out output
function CRC_Out= fcn(msg_raw)

divisor = 0x1D;
messageLength = 8;
CRC_raw = uint8(0x00);

for i = 1:length(msg_raw(:,1))

    message = bitxor(CRC_raw,msg_raw(i));

    for k = 1:messageLength
        if bitget(message,8)
            message = bitshift(message,1);
            message = bitxor(message,divisor);
        else
            message = bitshift(message,1);
        end
    end
    CRC_raw = message;

end

CRC_Out = bitxor(CRC_raw,0x00);

== stateflow chart halout/HAL_OUT/CAN3/FD3_VCU2_toNIDEC_Tx/Chart ==
  state TrigCounter
    en:
    counter = 0;
    counter++;
    (default) -> (junction 5)
    TrigCounter -> (junction 5) : {
        | counter++;
        | }
    (junction 5) -> (junction 6) [order 1] : [TxReq && (counter %% CycleCnt) == 0]
    (junction 5) -> (junction 7) [order 2]
    (junction 6) -> (junction 8) : {
        | TxTrigger;
        | counter = 0;
        | }
    (junction 8) -> (junction 7)
    (junction 7) -> (junction 34)
    (junction 34) -> (junction 33) [order 1] : [ !TxReq]
    (junction 34) -> (junction 35) [order 2]
    (junction 33) -> (junction 36) : {
        | counter = 0;
        | }
    (junction 36) -> (junction 35)
    (junction 35) -> (junction 44)
  data: TxReq input; CycleCnt input; counter local uint16
  events: TxTrigger output FUNCTION_CALL_EVENT

== matlab function halout/HAL_OUT/CAN3/FD3_VCU2_toNIDEC_0x154/CRC8_IfAction_Tx/If Action Subsystem/CRC8_Caculation/MATLAB Function ==
  data: msg_raw input; CRC_Out output
function CRC_Out= fcn(msg_raw)

divisor = 0x1D;
messageLength = 8;
CRC_raw = uint8(0xFF);

for i = 1:length(msg_raw(:,1))

    message = bitxor(CRC_raw,msg_raw(i));

    for k = 1:messageLength
        if bitget(message,8)
            message = bitshift(message,1);
            message = bitxor(message,divisor);
        else
            message = bitshift(message,1);
        end
    end
    CRC_raw = message;

end

CRC_Out = bitxor(CRC_raw,0xFF);

== matlab function halout/HAL_OUT/CAN3/FD3_VCU2_toNIDEC_0x154/CRC8_IfAction_Tx/If Action Subsystem1/CRC8_E2EProfile1/MATLAB Function ==
  data: msg_raw input; CRC_Out output
function CRC_Out= fcn(msg_raw)

divisor = 0x1D;
messageLength = 8;
CRC_raw = uint8(0x00);

for i = 1:length(msg_raw(:,1))

    message = bitxor(CRC_raw,msg_raw(i));

    for k = 1:messageLength
        if bitget(message,8)
            message = bitshift(message,1);
            message = bitxor(message,divisor);
        else
            message = bitshift(message,1);
        end
    end
    CRC_raw = message;

end

CRC_Out = bitxor(CRC_raw,0x00);

== stateflow chart halout/HAL_OUT/CAN4/FD4_CE100_0_Tx/Chart ==
  state TrigCounter
    en:
    counter = 0;
    counter++;
    (default) -> (junction 55) : {DelayWorkaround = 0;}
    TrigCounter -> (junction 55) : {
        | counter++;
        | CycleTriggerred = FALSE;
        | DelayWorkaround++;
        | }
    (junction 55) -> (junction 31) [order 2]
    (junction 55) -> (junction 5) [order 1] : [DelayWorkaround >= 0]{DelayWorkaround = 0;}
    (junction 5) -> (junction 6) [order 1] : [TxReq && (counter %% CycleCnt) == 0]
    (junction 5) -> (junction 7) [order 2]
    (junction 6) -> (junction 8) : {
        | TriggerDataUpdate;
        | TriggerCallCDD;
        | counter = 0;
        | CycleTriggerred =TRUE;
        | }
    (junction 8) -> (junction 7)
    (junction 7) -> (junction 34)
    (junction 34) -> (junction 38) [order 1] : [TxReq && EventReq && !CycleTriggerred]
    (junction 34) -> (junction 36) [order 2]
    (junction 38) -> (junction 40) : {
        | TriggerDataUpdate;
        | TriggerCallCDD;
        | }
    (junction 40) -> (junction 36)
    (junction 36) -> (junction 21)
    (junction 21) -> (junction 23) [order 1] : [ !TxReq]
    (junction 21) -> (junction 22) [order 2]
    (junction 23) -> (junction 20) : {
        | counter = 0;
        | }
    (junction 20) -> (junction 22)
    (junction 22) -> (junction 31)
  data: TxReq input; EventReq input; CycleCnt input; counter local uint16; CycleTriggerred local boolean; FALSE parameter; TRUE parameter; DelayWorkaround local double
  events: TriggerDataUpdate output FUNCTION_CALL_EVENT; TriggerCallCDD output FUNCTION_CALL_EVENT

== matlab function halout/HAL_OUT/CAN4/FD4_CE100_0_0x116/CRC8_IfAction_Tx/If Action Subsystem/CRC8_Caculation/MATLAB Function ==
  data: msg_raw input; CRC_Out output
function CRC_Out= fcn(msg_raw)

divisor = 0x1D;
messageLength = 8;
CRC_raw = uint8(0xFF);

for i = 1:length(msg_raw(:,1))

    message = bitxor(CRC_raw,msg_raw(i));

    for k = 1:messageLength
        if bitget(message,8)
            message = bitshift(message,1);
            message = bitxor(message,divisor);
        else
            message = bitshift(message,1);
        end
    end
    CRC_raw = message;

end

CRC_Out = bitxor(CRC_raw,0xFF);

== matlab function halout/HAL_OUT/CAN4/FD4_CE100_0_0x116/CRC8_IfAction_Tx/If Action Subsystem1/CRC8_E2EProfile1/MATLAB Function ==
  data: msg_raw input; CRC_Out output
function CRC_Out= fcn(msg_raw)

divisor = 0x1D;
messageLength = 8;
CRC_raw = uint8(0x00);

for i = 1:length(msg_raw(:,1))

    message = bitxor(CRC_raw,msg_raw(i));

    for k = 1:messageLength
        if bitget(message,8)
            message = bitshift(message,1);
            message = bitxor(message,divisor);
        else
            message = bitshift(message,1);
        end
    end
    CRC_raw = message;

end

CRC_Out = bitxor(CRC_raw,0x00);

== matlab function halout/HAL_OUT/CAN3/FD3_VCU2_0x153/CRC8_IfAction_Tx/If Action Subsystem/CRC8_Caculation/MATLAB Function ==
  data: msg_raw input; CRC_Out output
function CRC_Out= fcn(msg_raw)

divisor = 0x1D;
messageLength = 8;
CRC_raw = uint8(0xFF);

for i = 1:length(msg_raw(:,1))

    message = bitxor(CRC_raw,msg_raw(i));

    for k = 1:messageLength
        if bitget(message,8)
            message = bitshift(message,1);
            message = bitxor(message,divisor);
        else
            message = bitshift(message,1);
        end
    end
    CRC_raw = message;

end

CRC_Out = bitxor(CRC_raw,0xFF);
